simulink model "P4p2_integrator"  (R2014a)
settings: Solver=ode1  StartTime=0.0  StopTime=inf  FixedStep=0.002  RelTol=1e-3
PostLoadFcn:
  | qc_set_target_type(getConfigSet(bdroot, 'QUARC Default Target Configuration'));
values from neighbouring files (symbols this model uses):
  A_sys = [0 1 0 0 0 0; 0 0 0 0 0 0; 0 0 0 1 0 0; 0 0 0 0 0 0; 0 0 0 0 0 1; K_3 0 0 0 0 0]    [P4p2_integrator_init.m]    (also in P4p3_init.m; p4p2_NEW_test.m)
  B_sys = [0 0; 0 K_1; K_2 0; 0 0; 0 0; 0 0]    [P4p2_integrator_init.m]    (also in P4p3_init.m; p4p2_NEW_test.m)
  C_sys = [1 0 0 0 0 0; 0 0 1 0 0 0; 0 0 0 0 1 0]    [P4p2_integrator_init.m]    (also in P4p3_init.m = [0 0 1 0 0 0; 0 0 0 0 1 0]; p4p2_NEW_test.m)
  Joystick_gain_x = 1    [P4p2_integrator_init.m]    (also in P4p3_init.m; p4p2_NEW_test.m)
  Joystick_gain_y = -1    [P4p2_integrator_init.m]    (also in P4p3_init.m; p4p2_NEW_test.m)
  K_reg = lqr(A_reg, B_reg, Q_reg, R)    [P4p2_integrator_init.m]    (also in P4p3_init.m; p4p2_NEW_test.m)
  L = transpose(place(transpose(A_sys),transpose(C_sys),eigen))    [P4p2_integrator_init.m]    (also in P4p3_init.m; p4p2_NEW_test.m)
  P = -(C_reg*((A_reg_cut-B_reg_cut*K_reg_cut)^(-1))*B_reg_cut)^(-1)    [P4p2_integrator_init.m]    (also in P4p3_init.m; p4p2_NEW_test.m = -(C_reg*((A_reg-B_reg*K_reg)^(-1))*B_reg)^(-1))
undefined symbols (not defined in the file or in its folder): HIL, qc_get_step_size
libraries: simulink_extras x6, quarc_library x4
settings Model: SimulationMode=external  ExtModeTrigDuration=5000  Creator=Rchan  LastModifiedBy=sondrehf
settings SolverCC: PositivePriorityOrder=on
settings DataIOCC: SignalLoggingSaveFormat=ModelDataLogs
settings OptimizationCC: ExpressionDepthLimit=2147483647  InitFltsAndDblsToZero=on
settings DebuggingCC: SaveWithParameterizedLinksMsg=none  UnderspecifiedInitializationDetection=Classic  MultiTaskDSMMsg=warning  MultiTaskCondExecSysMsg=none  FcnCallInpInsideContextMsg=UseLocalSettings  StateNameClashWarn=warning
settings RTWCC: SystemTargetFile=quarc_win64.tlc  TemplateMakefile=quarc_default_tmf  Description=QUARC Win64 Target  ProcessScript=quarc_win64_make_rtw_hook
settings STFCustomTargetCC: CPPClassGenCompliant=on
settings GRTTargetCC: ParMdlRefBuildCompliant=off  CompOptLevelCompliant=off  CombineOutputUpdateFcns=off  MatFileLogging=off  GRTInterface=on  ExtMode=on  ExtModeMexFile=quarc_comm

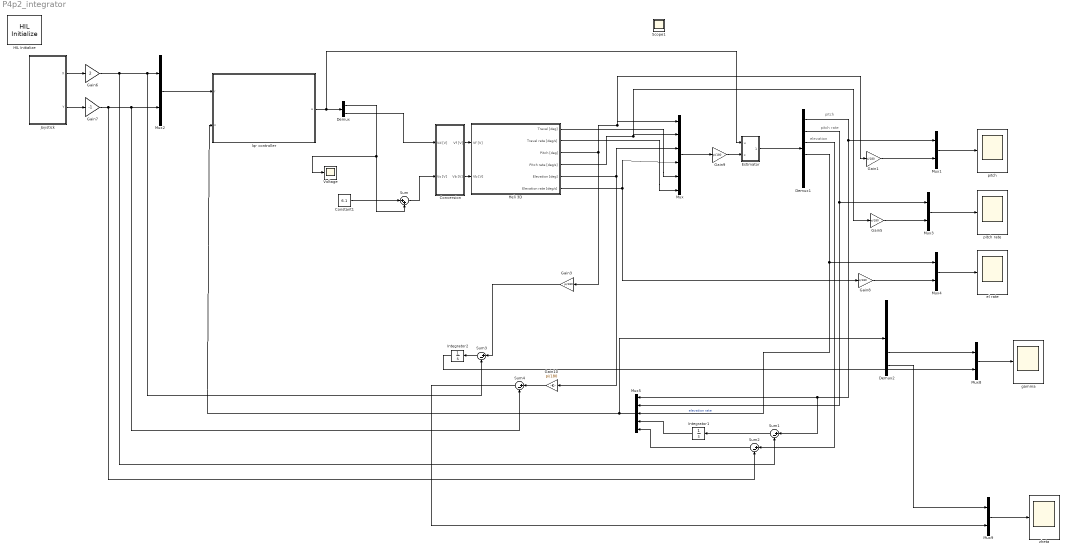
== system P4p2_integrator ==
  note: elevation
  note: pitch rate
  note: pitch
  Constant1 : Constant  Value=6.1
  Conversion : Subsystem
  Demux : Demux  Outputs=2
  Demux1 : Demux  Outputs=6
  Demux2 : Demux  Outputs=5
  "Estimator " : Subsystem
  Gain{1,3,5,8..10} (6 alike) : Gain  Gain=pi/180
  Gain6 : Gain  Gain=2
  Gain7 : Gain  Gain=-1
  HIL Initialize : quarc_library/Data Acquisition/Generic/Configuration/HIL Initialize  Priority=-99  object_name=HIL-1  board_type=q8_usb  board_number=0  board_options=update_rate=normal;decimation=1  exclusive=off  active=off  hardware_clocks=[0:2]  clock_modes=[]  initial_clock_frequencies=[]  set_clock_params_at_start=off  set_clock_params_at_switch_in=off  set_clock_frequencies_at_start=off  set_clock_frequencies_at_switch_in=off  analog_input_channels=[0:7]  analog_input_maximums=10  analog_input_minimums=-10  set_analog_input_params_at_start=on  set_analog_input_params_at_switch_in=off  analog_output_channels=[0:7]  analog_output_maximums=10  analog_output_minimums=-10  initial_analog_outputs=[0]  final_analog_outputs=[0]  watchdog_analog_outputs=0  set_analog_output_params_at_start=on  set_analog_output_params_at_switch_in=off  set_analog_outputs_at_start=on  set_analog_outputs_at_switch_in=off  set_analog_outputs_at_terminate=on  set_analog_outputs_at_switch_out=off  set_analog_outputs_on_watchdog=off  digital_input_channels=[]  digital_output_channels=[]  digital_output_configuration=[]  initial_digital_outputs=[1]  final_digital_outputs=[1]  watchdog_digital_outputs=[1]  set_digital_output_params_at_start=off  set_digital_output_params_at_switch_in=off  set_digital_outputs_at_start=on  set_digital_outputs_at_switch_in=off  set_digital_outputs_at_terminate=on  set_digital_outputs_at_switch_out=off  set_digital_outputs_on_watchdog=off  encoder_channels=[0:7]  quadrature=[4]  encoder_filter_frequency=[]  initial_encoder_counts=[0]  set_encoder_params_at_start=on  set_encoder_params_at_switch_in=off  set_encoder_counts_at_start=on  set_encoder_counts_at_switch_in=off  pwm_channels=[0:7]  pwm_modes=0  pwm_frequency=99.532799999999995e6/4095  pwm_configuration=[0]  pwm_alignment=[0]  pwm_polarity=[1]  pwm_leading_deadband=[0]  pwm_trailing_deadband=[0]  initial_pwm_outputs=[0]  final_pwm_outputs=[0]  watchdog_pwm_outputs=[0]  set_pwm_params_at_start=on  set_pwm_params_at_switch_in=off  set_pwm_outputs_at_start=on  set_pwm_outputs_at_switch_in=off  set_pwm_outputs_at_terminate=on  set_pwm_outputs_at_switch_out=off  set_pwm_outputs_on_watchdog=off  other_output_channels=[]  initial_other_outputs=[]  final_other_outputs=[]  watchdog_other_outputs=[]  set_other_outputs_at_start=off  set_other_outputs_at_switch_in=off  set_other_outputs_at_terminate=off  set_other_outputs_at_switch_out=off  set_other_outputs_on_watchdog=off
  Heli 3D : Subsystem
  Integrator1 : Integrator
  Integrator2 : Integrator
  Joystick : Subsystem
  Mux : Mux  Inputs=6
  Mux{1..4,8..9} (6 alike) : Mux  Inputs=2
  Mux5 : Mux  Inputs=5
  Scope1 : Scope
      settings: TimeRange=40  YMin=-25  YMax=40  SaveName=ScopeData4
  Sum : Sum  Inputs=|++
  Sum{1..4} (4 alike) : Sum  Inputs=|+-
  Voltage : Scope
      settings: TimeRange=40  YMin=-25  YMax=40  SaveName=ScopeData6
  el rate : Scope
      settings: TimeRange=10  YMin=-32.5  SaveName=ScopeData15
  "gamma " : Scope
      settings: YMin=-1  YMax=0.8  SaveName=ScopeData16
  lqr controller : Subsystem
  pitch : Scope
      settings: SaveName=ScopeData14
  pitch rate : Scope
      settings: YMin=-2  YMax=2.25  SaveName=ScopeData17
  zheta : Scope
      settings: YMin=-25  YMax=30  SaveName=ScopeData18
  wires:
  Conversion/2(Vb [V]) -> Heli 3D/2(Vb [V])
  Conversion/1(Vf [V]) -> Heli 3D/1(Vf [V])
  Sum/1 -> Conversion/2(Vs [V])
  Joystick/1(X) -> Gain6/1
  Joystick/2(Y) -> Gain7/1
  Demux/1 -> Sum/2, Voltage/1
  lqr controller/1("u ") -> "Estimator "/1(u), Demux/1
  Demux/2 -> Conversion/1(Vd [V])
  Constant1/1 -> Sum/1
  Mux/1 -> Gain9/1
  Gain9/1 -> "Estimator "/2("x ")
  Mux2/1 -> lqr controller/1(r)
  "Estimator "/1("x_hat ") -> Demux1/1
  Mux1/1 -> pitch/1
  Mux3/1 -> pitch rate/1
  Mux4/1 -> el rate/1
  Heli 3D/5(Elevation [deg]) -> Gain10/1, Mux/3
  Heli 3D/1(Travel [deg]) -> Mux/5
  Heli 3D/2(Travel rate [deg/s]) -> Mux/6
  Demux1/1 -> Mux1/1, Sum1/1, Mux5/1
  Demux1/2 -> Mux3/1, Mux5/2
  Demux1/4 -> Mux4/1, Mux5/3  "elevation rate"
  Sum1/1 -> Integrator1/1
  Sum2/1 -> Mux5/5
  Heli 3D/4(Pitch rate [deg/s]) -> Mux/2, Gain5/1
  Heli 3D/6(Elevation rate [deg/s]) -> Gain8/1, Mux/4
  Gain6/1 -> Sum3/2, Mux2/1, Sum1/2
  Gain7/1 -> Mux2/2, Sum4/2, Sum2/2
  Gain3/1 -> Sum3/1
  Heli 3D/3(Pitch [deg]) -> Gain3/1, Mux/1, Gain1/1
  Sum3/1 -> Integrator2/1
  Sum4/1 -> Mux9/2
  Integrator2/1 -> Mux8/2
  Mux8/1 -> "gamma "/1
  Mux9/1 -> zheta/1
  Gain1/1 -> Mux1/2
  Gain5/1 -> Mux3/2
  Gain8/1 -> Mux4/2
  Integrator1/1 -> Mux5/4
  Demux2/4 -> Mux8/1
  Demux1/3 -> Sum2/1
  Demux2/5 -> Mux9/1
  Gain10/1 -> Sum4/1
  Mux5/1 -> lqr controller/2(x), Demux2/1

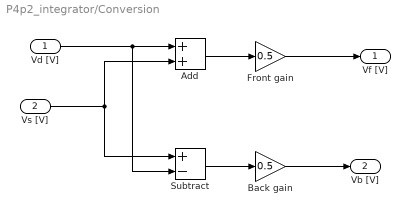
== system P4p2_integrator/Conversion ==
  Vd [V] : Inport
  Vs [V] : Inport  Port=2
  Add : Sum
  Back gain : Gain  Gain=0.5
  Front gain : Gain  Gain=0.5
  Subtract : Sum  Inputs=+-
  Vf [V] : Outport
  Vb [V] : Outport  Port=2
  wires:
  Vd [V]/1 -> Subtract/2, Add/1
  Vs [V]/1 -> Subtract/1, Add/2
  Subtract/1 -> Back gain/1
  Back gain/1 -> Vb [V]/1
  Add/1 -> Front gain/1
  Front gain/1 -> Vf [V]/1

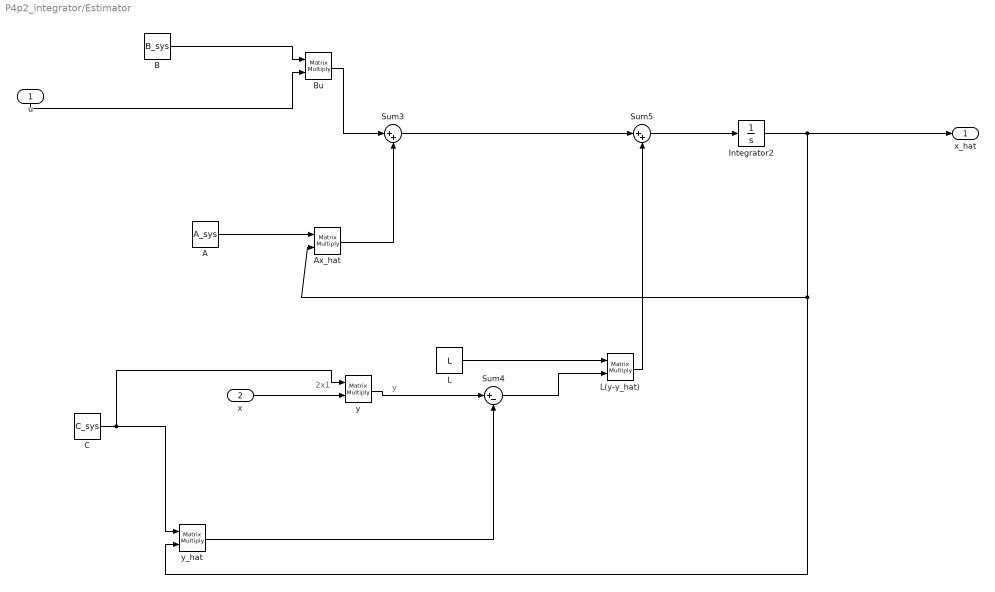
== system P4p2_integrator/Estimator  ==
  note: 2x1
  note: y
  u : Inport
  "x " : Inport  Port=2
  A : Constant  Value=A_sys
  Ax_hat : Product  Multiplication=Matrix(*)
  B : Constant  Value=B_sys
  Bu : Product  Multiplication=Matrix(*)
  C : Constant  Value=C_sys
  Integrator2 : Integrator
  L : Constant  Value=L
  L(y-y_hat) : Product  Multiplication=Matrix(*)
  Sum3 : Sum  Inputs=|++
  Sum4 : Sum  Inputs=|+-
  Sum5 : Sum  Inputs=|++
  y : Product  Multiplication=Matrix(*)
  y_hat : Product  Multiplication=Matrix(*)
  "x_hat " : Outport
  wires:
  Integrator2/1 -> Ax_hat/2, y_hat/2, "x_hat "/1
  Ax_hat/1 -> Sum3/2
  u/1 -> Bu/2
  C/1 -> y_hat/1, y/1
  y_hat/1 -> Sum4/2
  B/1 -> Bu/1
  A/1 -> Ax_hat/1
  y/1 -> Sum4/1
  L/1 -> L(y-y_hat)/1
  Sum4/1 -> L(y-y_hat)/2
  Bu/1 -> Sum3/1
  Sum3/1 -> Sum5/1
  Sum5/1 -> Integrator2/1
  L(y-y_hat)/1 -> Sum5/2
  "x "/1 -> y/2

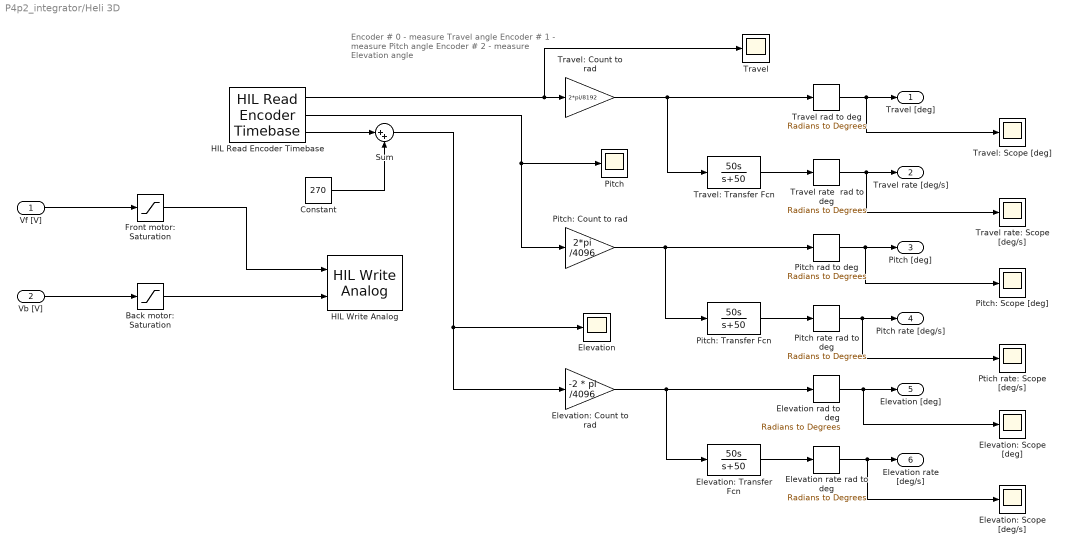
== system P4p2_integrator/Heli 3D ==
  note: Encoder # 0 - measure Travel angle
      | Encoder # 1 - measure Pitch angle
      | Encoder # 2 - measure Elevation angle
  Vf [V] : Inport
  Vb [V] : Inport  Port=2
  Back motor: Saturation : Saturate  UpperLimit=5  LowerLimit=-5
  Constant : Constant  Value=270
  Elevation : Scope
      settings: YMin=-50  YMax=300  SaveName=ScopeData2
  Elevation rad to deg : simulink_extras/Transformations/Radians to Degrees
  Elevation rate rad to deg : simulink_extras/Transformations/Radians to Degrees
  Elevation: Count to rad : Gain  Gain=-2 * pi /4096
  Elevation: Scope [deg/s] : Scope
      settings: YMin=-15  YMax=15  SaveName=ScopeData13
  Elevation: Scope [deg] : Scope
      settings: YMin=-30  YMax=40  SaveName=ScopeData12
  Elevation: Transfer Fcn : TransferFcn  Numerator=[50 0]  Denominator=[1 50]
  Front motor: Saturation : Saturate  UpperLimit=5  LowerLimit=-5
  HIL Read Encoder Timebase : quarc_library/Data Acquisition/Generic/Timebases/HIL Read Encoder Timebase  object_name=HIL-1  clock=0  channels=[0:2]  samples_in_buffer=max(ceil(1/qc_get_step_size), 1)  active=on  vector_output=off  data_type_mode=Inherit via back propagation  data_type=double
  HIL Write Analog : quarc_library/Data Acquisition/Generic/Immediate I//O/HIL Write Analog  object_name=HIL-1  channels=[0:1]  sample_time=-1  active=off  vector_input=off
  "Pitch " : Scope
      settings: YMin=-300  YMax=500
  Pitch rad to deg : simulink_extras/Transformations/Radians to Degrees
  Pitch rate rad to deg : simulink_extras/Transformations/Radians to Degrees
  Pitch: Count to rad : Gain  Gain=2*pi /4096
  Pitch: Scope [deg] : Scope
      settings: YMin=-25  YMax=32.5  SaveName=ScopeData10
  Pitch: Transfer Fcn : TransferFcn  Numerator=[50 0]  Denominator=[1 50]
  Ptich rate: Scope [deg/s] : Scope
      settings: YMin=-15  YMax=15  SaveName=ScopeData11
  Sum : Sum  Inputs=|++
  "Travel " : Scope
      settings: YMin=-1000  YMax=2250
  Travel rad to deg : simulink_extras/Transformations/Radians to Degrees
  Travel rate  rad to deg : simulink_extras/Transformations/Radians to Degrees
  Travel rate: Scope [deg/s] : Scope
      settings: YMin=-30  YMax=40  SaveName=ScopeData9
  Travel: Count to rad : Gain  Gain=2*pi/8192
  Travel: Scope [deg] : Scope
      settings: YMin=-17  YMax=0  SaveName=ScopeData8
  Travel: Transfer Fcn : TransferFcn  Numerator=[50 0]  Denominator=[1 50]
  Travel [deg] : Outport
  Travel rate [deg/s] : Outport  Port=2
  Pitch [deg] : Outport  Port=3
  Pitch rate [deg/s] : Outport  Port=4
  Elevation [deg] : Outport  Port=5
  Elevation rate [deg/s] : Outport  Port=6
  wires:
  HIL Read Encoder Timebase/1 -> "Travel "/1, Travel: Count to rad/1
  HIL Read Encoder Timebase/2 -> "Pitch "/1, Pitch: Count to rad/1
  HIL Read Encoder Timebase/3 -> Sum/1
  Travel: Count to rad/1 -> Travel: Transfer Fcn/1, Travel rad to deg/1
  Travel: Transfer Fcn/1 -> Travel rate  rad to deg/1
  Pitch: Count to rad/1 -> Pitch: Transfer Fcn/1, Pitch rad to deg/1
  Pitch: Transfer Fcn/1 -> Pitch rate rad to deg/1
  Elevation: Count to rad/1 -> Elevation: Transfer Fcn/1, Elevation rad to deg/1
  Elevation: Transfer Fcn/1 -> Elevation rate rad to deg/1
  Travel rad to deg/1 -> Travel: Scope [deg]/1, Travel [deg]/1
  Travel rate  rad to deg/1 -> Travel rate: Scope [deg/s]/1, Travel rate [deg/s]/1
  Pitch rad to deg/1 -> Pitch: Scope [deg]/1, Pitch [deg]/1
  Pitch rate rad to deg/1 -> Ptich rate: Scope [deg/s]/1, Pitch rate [deg/s]/1
  Elevation rad to deg/1 -> Elevation: Scope [deg]/1, Elevation [deg]/1
  Elevation rate rad to deg/1 -> Elevation: Scope [deg/s]/1, Elevation rate [deg/s]/1
  Vf [V]/1 -> Front motor: Saturation/1
  Vb [V]/1 -> Back motor: Saturation/1
  Front motor: Saturation/1 -> HIL Write Analog/1
  Back motor: Saturation/1 -> HIL Write Analog/2
  Sum/1 -> Elevation/1, Elevation: Count to rad/1
  Constant/1 -> Sum/2

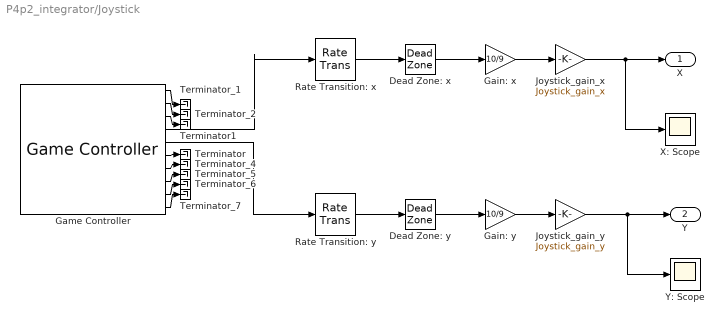
== system P4p2_integrator/Joystick ==
  Dead Zone: x : DeadZone  LowerValue=-0.1  UpperValue=0.1  SaturateOnIntegerOverflow=on
  Dead Zone: y : DeadZone  LowerValue=-0.1  UpperValue=0.1  SaturateOnIntegerOverflow=on
  Gain: x : Gain  Gain=10/9
  Gain: y : Gain  Gain=10/9
  Game Controller : quarc_library/Devices/Peripherals/Target/Game Controller  controller=1  buffer_size=12  deadzone=[]  saturation=[]  sample_time=max(qc_get_step_size, 0.01)  auto_center=off  enabled=on
  Joystick_gain_x : Gain  Gain=Joystick_gain_x
  Joystick_gain_y : Gain  Gain=Joystick_gain_y
  Rate Transition: x : RateTransition
  Rate Transition: y : RateTransition
  Terminator : Terminator
  Terminator1 : Terminator
  Terminator_{1..2,4..7} (6 alike) : Terminator
  X: Scope : Scope
      settings: YMin=-1  YMax=1  SaveName=ScopeData7
  Y: Scope : Scope
      settings: YMin=-10  YMax=10  SaveName=ScopeData5
  X : Outport
  Y : Outport  Port=2
  wires:
  Rate Transition: y/1 -> Dead Zone: y/1
  Rate Transition: x/1 -> Dead Zone: x/1
  Game Controller/5 -> Rate Transition: y/1
  Game Controller/4 -> Rate Transition: x/1
  Game Controller/1 -> Terminator_1/1
  Game Controller/2 -> Terminator_2/1
  Game Controller/7 -> Terminator_4/1
  Game Controller/8 -> Terminator_5/1
  Game Controller/9 -> Terminator_6/1
  Game Controller/10 -> Terminator_7/1
  Game Controller/3 -> Terminator1/1
  Game Controller/6 -> Terminator/1
  Dead Zone: x/1 -> Gain: x/1
  Dead Zone: y/1 -> Gain: y/1
  Gain: x/1 -> Joystick_gain_x/1
  Gain: y/1 -> Joystick_gain_y/1
  Joystick_gain_x/1 -> X/1, X: Scope/1
  Joystick_gain_y/1 -> Y: Scope/1, Y/1

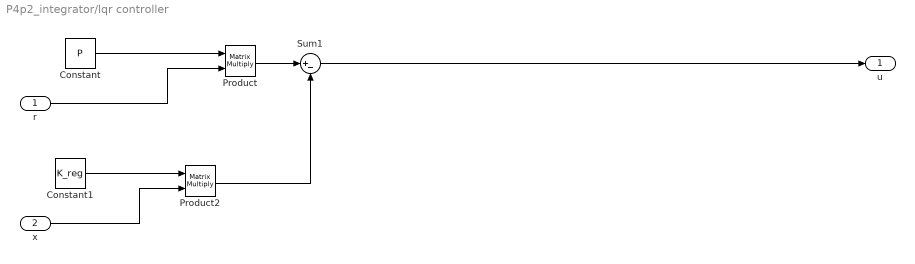
== system P4p2_integrator/lqr controller ==
  r : Inport
  x : Inport  Port=2
  Constant : Constant  Value=P
  Constant1 : Constant  Value=K_reg
  Product : Product  Multiplication=Matrix(*)
  Product2 : Product  Multiplication=Matrix(*)
  Sum1 : Sum  Inputs=|+-
  "u " : Outport
  wires:
  Product/1 -> Sum1/1
  x/1 -> Product2/2
  Product2/1 -> Sum1/2
  Sum1/1 -> "u "/1
  Constant1/1 -> Product2/1
  Constant/1 -> Product/1
  r/1 -> Product/2
